simulink model "sm_aileron_actuator_mech_01_ail"  (R2026a)
settings: Solver=VariableStepAuto  EnableMultiTasking=on
PreLoadFcn:
  | aileronAssembly_DataFile
undefined symbols (not defined in the file): AAC_Param, actbase_x, actbase_y, smiData, X, Y, Z
libraries: sm_lib x303, nesl_utility x1
(part 2 of 6)

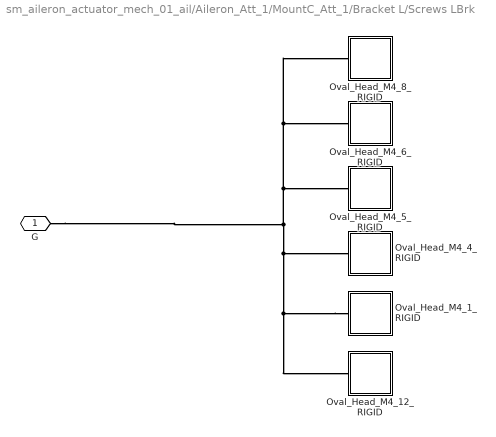
== system sm_aileron_actuator_mech_01_ail/Aileron_Att_1/MountC_Att_1/Bracket L/Screws LBrk ==
  Oval_Head_M4_12_RIGID : Subsystem  RequirementInfo={} %GIDa_408545e4_969e_4b12_8d49_3ebac226240b
  Oval_Head_M4_1_RIGID : Subsystem  RequirementInfo={} %GIDa_fd160c21_93a2_41e0_88bc_776c68d5a1b4
  Oval_Head_M4_4_RIGID : Subsystem  RequirementInfo={} %GIDa_6f4e9814_9943_43be_96b6_78b1aff6dd74
  Oval_Head_M4_5_RIGID : Subsystem  RequirementInfo={} %GIDa_7c459a83_8431_46f1_9d88_31310de40f59
  Oval_Head_M4_6_RIGID : Subsystem  RequirementInfo={} %GIDa_d922eb42_8b80_410e_876a_99bf2bbe6032
  Oval_Head_M4_8_RIGID : Subsystem  RequirementInfo={} %GIDa_ea3f8b8a_bed4_4299_99e1_7a89c2fafe6f
  G : PMIOPort  RequirementInfo={} %GIDa_d90268cf_c8b4_4cb9_9e17_a6888775eb52  Side=Left
  connections:
  Oval_Head_M4_1_RIGID/LConn1 -- G/RConn1 -- Oval_Head_M4_8_RIGID/LConn1 -- Oval_Head_M4_6_RIGID/LConn1 -- Oval_Head_M4_5_RIGID/LConn1 -- Oval_Head_M4_4_RIGID/LConn1 -- Oval_Head_M4_12_RIGID/LConn1

== system sm_aileron_actuator_mech_01_ail/Aileron_Att_1/MountC_Att_1/Bracket R/AilBrk_R_1_RIGID ==
  ReferenceFrame : sm_lib/Frames and Transforms/Reference Frame  RequirementInfo={} %GIDa_74c56975_f3eb_4fd4_b567_ce3850dcc004
  Solid : sm_lib/Body Elements/File Solid  RequirementInfo={} %GIDa_802e2630_df3e_46c3_94a4_2f58f44522fa  ExtGeomFileName=AilBrk_R.step  UnitType=FromFile  ExtGeomFileUnits=m  StepReaderType=HEX  ExportConvexHullGeometry=off  InertiaType=Custom  BasedOnType=Density  Density=1000  DensityUnits=kg/m^3  Mass=smiData.Solid(16).mass  MassUnits=kg  CenterOfMass=smiData.Solid(16).CoM  CenterOfMassUnits=m  MomentsOfInertia=smiData.Solid(16).MoI  MomentsOfInertiaUnits=kg*m^2  ProductsOfInertia=smiData.Solid(16).PoI  ProductsOfInertiaUnits=kg*m^2  GraphicType=FromGeometry  MarkerShape=Sphere  MarkerSize=10  GraphicVisPropType=SimpleVisualProperties  GraphicDiffuseColor=smiData.Solid(16).color  GraphicOpacity=smiData.Solid(16).opacity  GraphicSpecularColor=[0.5 0.5 0.5 1.0]  GraphicAmbientColor=[0.15 0.15 0.15 1.0]  GraphicEmissiveColor=[0.0 0.0 0.0 1.0]  GraphicShininess=75  DoExposeReferenceFrame=on  SerializedFrames=<Frames/>
  Transform : sm_lib/Frames and Transforms/Rigid Transform  RequirementInfo={} %GIDa_83aa15e3_dddf_412e_ac7a_0a1ce9ef137c  RotationMethod=ArbitraryAxis  FollAlignAxisA=+X  BaseAlignAxisA=+Y  FollAlignAxisB=+Y  BaseAlignAxisB=+Z  RotationStandardAxis=+Z  RotationAngle=smiData.RigidTransform(82).angle  RotationAngleUnits=rad  RotationArbitraryAxis=smiData.RigidTransform(82).axis  RotationSequenceAxes=FollowerAxes  RotationSequence=XYX  RotationSequenceAngles=[0 0 0]  RotationSequenceAnglesUnits=deg  RotationMatrix=[1 0 0; 0 1 0; 0 0 1]  Quaternion=[1 0 0 0]  TranslationMethod=Cartesian  TranslationCartesianOffset=smiData.RigidTransform(82).translation  TranslationCartesianOffsetUnits=m  TranslationStandardAxis=+Z  TranslationStandardOffset=0  TranslationStandardOffsetUnits=m  TranslationROffset=0  TranslationROffsetUnits=m  TranslationThetaOffset=0  TranslationThetaOffsetUnits=deg  TranslationZOffset=0  TranslationZOffsetUnits=m
  Transform Manual4Vis : sm_lib/Frames and Transforms/Rigid Transform  RequirementInfo={} %GIDa_283d4460_364a_4cfb_ae13_3c69dcaaddcc  RotationMethod=None  FollAlignAxisA=+X  BaseAlignAxisA=+Y  FollAlignAxisB=+Y  BaseAlignAxisB=+Z  RotationStandardAxis=+Z  RotationAngle=0.0  RotationAngleUnits=deg  RotationArbitraryAxis=[0 0 1]  RotationSequenceAxes=FollowerAxes  RotationSequence=XYX  RotationSequenceAngles=[0 0 0]  RotationSequenceAnglesUnits=deg  RotationMatrix=[1 0 0; 0 1 0; 0 0 1]  Quaternion=[1 0 0 0]  TranslationMethod=StandardAxis  TranslationCartesianOffset=[0 0 0]  TranslationCartesianOffsetUnits=m  TranslationStandardAxis=-Y  TranslationStandardOffset=AAC_Param.AilBrk.LRManual4Vis  TranslationStandardOffsetUnits=m  TranslationROffset=0  TranslationROffsetUnits=m  TranslationThetaOffset=0  TranslationThetaOffsetUnits=deg  TranslationZOffset=0  TranslationZOffsetUnits=m
  Transform1 : sm_lib/Frames and Transforms/Rigid Transform  RequirementInfo={} %GIDa_a1c92bec_f7fd_44f1_b946_6fd160cd1aa4  RotationMethod=ArbitraryAxis  FollAlignAxisA=+X  BaseAlignAxisA=+Y  FollAlignAxisB=+Y  BaseAlignAxisB=+Z  RotationStandardAxis=+Z  RotationAngle=smiData.RigidTransform(176).angle  RotationAngleUnits=rad  RotationArbitraryAxis=smiData.RigidTransform(176).axis  RotationSequenceAxes=FollowerAxes  RotationSequence=XYX  RotationSequenceAngles=[0 0 0]  RotationSequenceAnglesUnits=deg  RotationMatrix=[1 0 0; 0 1 0; 0 0 1]  Quaternion=[1 0 0 0]  TranslationMethod=Cartesian  TranslationCartesianOffset=smiData.RigidTransform(176).translation  TranslationCartesianOffsetUnits=m  TranslationStandardAxis=+Z  TranslationStandardOffset=0  TranslationStandardOffsetUnits=m  TranslationROffset=0  TranslationROffsetUnits=m  TranslationThetaOffset=0  TranslationThetaOffsetUnits=deg  TranslationZOffset=0  TranslationZOffsetUnits=m
  G : PMIOPort  RequirementInfo={} %GIDa_d384faa3_ef63_4569_b23e_5e858ec3c873  Side=Left
  F : PMIOPort  RequirementInfo={} %GIDa_a6f33151_7075_4140_acee_fcb6192613cb  Port=2  Side=Right
  connections:
  Transform Manual4Vis/LConn1 -- ReferenceFrame/RConn1 -- Transform1/LConn1 -- Transform/RConn1
  Transform/LConn1 -- G/RConn1
  Transform1/RConn1 -- F/RConn1
  Transform Manual4Vis/RConn1 -- Solid/RConn1

== system sm_aileron_actuator_mech_01_ail/Aileron_Att_1/MountC_Att_1/Bracket R/Bolt RBrk ==
  Hex_Bolt_M10_1_RIGID : Subsystem  RequirementInfo={} %GIDa_51443a49_e410_4c6d_a840_81d676008002
  Washer_2_RIGID : Subsystem  RequirementInfo={} %GIDa_85bd74db_0059_4442_b071_fa5b0071d56b
  G : PMIOPort  RequirementInfo={} %GIDa_2cce0c68_3112_45a6_92fd_f121ce5f1707  Side=Left
  connections:
  Hex_Bolt_M10_1_RIGID/LConn1 -- G/RConn1 -- Washer_2_RIGID/LConn1

== system sm_aileron_actuator_mech_01_ail/Aileron_Att_1/MountC_Att_1/Bracket R/Screws RBrk ==
  Oval_Head_M4_10_RIGID : Subsystem  RequirementInfo={} %GIDa_d0d1d250_6a18_49bc_9058_b5b8dcd1b587
  Oval_Head_M4_11_RIGID : Subsystem  RequirementInfo={} %GIDa_1e18def3_4770_457a_b532_f3b10f3dd7ac
  Oval_Head_M4_2_RIGID : Subsystem  RequirementInfo={} %GIDa_434c022c_7618_4f4a_9cd7_ab87bc38975f
  Oval_Head_M4_3_RIGID : Subsystem  RequirementInfo={} %GIDa_57ddbddc_0d8f_4cec_bf5d_8c5a1e167ae3
  Oval_Head_M4_7_RIGID : Subsystem  RequirementInfo={} %GIDa_79914485_e7cc_41fb_90bc_5dca6c20becd
  Oval_Head_M4_9_RIGID : Subsystem  RequirementInfo={} %GIDa_ea88f9c1_5feb_464a_844f_15d140c7da09
  G : PMIOPort  RequirementInfo={} %GIDa_a28f78b5_595c_4617_9aa7_5b39891ac86f  Side=Left
  connections:
  Oval_Head_M4_3_RIGID/LConn1 -- G/RConn1 -- Oval_Head_M4_10_RIGID/LConn1 -- Oval_Head_M4_11_RIGID/LConn1 -- Oval_Head_M4_2_RIGID/LConn1 -- Oval_Head_M4_9_RIGID/LConn1 -- Oval_Head_M4_7_RIGID/LConn1

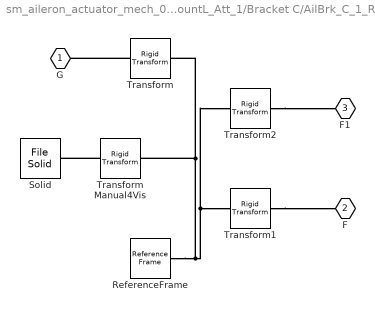
== system sm_aileron_actuator_mech_01_ail/Aileron_Att_1/MountL_Att_1/Bracket C/AilBrk_C_1_RIGID ==
  ReferenceFrame : sm_lib/Frames and Transforms/Reference Frame  RequirementInfo={} %GIDa_a871696a_d055_4df2_9121_142ef3f09b37
  Solid : sm_lib/Body Elements/File Solid  RequirementInfo={} %GIDa_5a36d86e_9075_441a_b790_2426bf56c7da  ExtGeomFileName=AilBrk_C.step  UnitType=FromFile  ExtGeomFileUnits=m  StepReaderType=HEX  ExportConvexHullGeometry=off  InertiaType=Custom  BasedOnType=Density  Density=1000  DensityUnits=kg/m^3  Mass=smiData.Solid(15).mass  MassUnits=kg  CenterOfMass=smiData.Solid(15).CoM  CenterOfMassUnits=m  MomentsOfInertia=smiData.Solid(15).MoI  MomentsOfInertiaUnits=kg*m^2  ProductsOfInertia=smiData.Solid(15).PoI  ProductsOfInertiaUnits=kg*m^2  GraphicType=FromGeometry  MarkerShape=Sphere  MarkerSize=10  GraphicVisPropType=SimpleVisualProperties  GraphicDiffuseColor=smiData.Solid(15).color  GraphicOpacity=smiData.Solid(15).opacity  GraphicSpecularColor=[0.5 0.5 0.5 1.0]  GraphicAmbientColor=[0.15 0.15 0.15 1.0]  GraphicEmissiveColor=[0.0 0.0 0.0 1.0]  GraphicShininess=75  DoExposeReferenceFrame=on  SerializedFrames=<Frames/>
  Transform : sm_lib/Frames and Transforms/Rigid Transform  RequirementInfo={} %GIDa_bf2783ef_b105_4d78_871d_57743bb0bee2  RotationMethod=ArbitraryAxis  FollAlignAxisA=+X  BaseAlignAxisA=+Y  FollAlignAxisB=+Y  BaseAlignAxisB=+Z  RotationStandardAxis=+Z  RotationAngle=smiData.RigidTransform(161).angle  RotationAngleUnits=rad  RotationArbitraryAxis=smiData.RigidTransform(161).axis  RotationSequenceAxes=FollowerAxes  RotationSequence=XYX  RotationSequenceAngles=[0 0 0]  RotationSequenceAnglesUnits=deg  RotationMatrix=[1 0 0; 0 1 0; 0 0 1]  Quaternion=[1 0 0 0]  TranslationMethod=Cartesian  TranslationCartesianOffset=smiData.RigidTransform(161).translation  TranslationCartesianOffsetUnits=m  TranslationStandardAxis=+Z  TranslationStandardOffset=0  TranslationStandardOffsetUnits=m  TranslationROffset=0  TranslationROffsetUnits=m  TranslationThetaOffset=0  TranslationThetaOffsetUnits=deg  TranslationZOffset=0  TranslationZOffsetUnits=m
  Transform Manual4Vis : sm_lib/Frames and Transforms/Rigid Transform  RequirementInfo={} %GIDa_31586e81_9f9a_4547_bcb3_9e99a8f792ea  RotationMethod=None  FollAlignAxisA=+X  BaseAlignAxisA=+Y  FollAlignAxisB=+Y  BaseAlignAxisB=+Z  RotationStandardAxis=+Z  RotationAngle=0.0  RotationAngleUnits=deg  RotationArbitraryAxis=[0 0 1]  RotationSequenceAxes=FollowerAxes  RotationSequence=XYX  RotationSequenceAngles=[0 0 0]  RotationSequenceAnglesUnits=deg  RotationMatrix=[1 0 0; 0 1 0; 0 0 1]  Quaternion=[1 0 0 0]  TranslationMethod=Cartesian  TranslationCartesianOffset=[-1 1 0]*AAC_Param.AilBrk.LRManual4Vis  TranslationCartesianOffsetUnits=m  TranslationStandardAxis=+Z  TranslationStandardOffset=0  TranslationStandardOffsetUnits=m  TranslationROffset=0  TranslationROffsetUnits=m  TranslationThetaOffset=0  TranslationThetaOffsetUnits=deg  TranslationZOffset=0  TranslationZOffsetUnits=m
  Transform1 : sm_lib/Frames and Transforms/Rigid Transform  RequirementInfo={} %GIDa_71a8cba1_f9af_4bc8_a1c0_4002b6347aec  RotationMethod=ArbitraryAxis  FollAlignAxisA=+X  BaseAlignAxisA=+Y  FollAlignAxisB=+Y  BaseAlignAxisB=+Z  RotationStandardAxis=+Z  RotationAngle=smiData.RigidTransform(185).angle  RotationAngleUnits=rad  RotationArbitraryAxis=smiData.RigidTransform(185).axis  RotationSequenceAxes=FollowerAxes  RotationSequence=XYX  RotationSequenceAngles=[0 0 0]  RotationSequenceAnglesUnits=deg  RotationMatrix=[1 0 0; 0 1 0; 0 0 1]  Quaternion=[1 0 0 0]  TranslationMethod=Cartesian  TranslationCartesianOffset=smiData.RigidTransform(185).translation  TranslationCartesianOffsetUnits=m  TranslationStandardAxis=+Z  TranslationStandardOffset=0  TranslationStandardOffsetUnits=m  TranslationROffset=0  TranslationROffsetUnits=m  TranslationThetaOffset=0  TranslationThetaOffsetUnits=deg  TranslationZOffset=0  TranslationZOffsetUnits=m
  Transform2 : sm_lib/Frames and Transforms/Rigid Transform  RequirementInfo={} %GIDa_2e2375df_b38c_4b24_9016_3885bd582684  RotationMethod=ArbitraryAxis  FollAlignAxisA=+X  BaseAlignAxisA=+Y  FollAlignAxisB=+Y  BaseAlignAxisB=+Z  RotationStandardAxis=+Z  RotationAngle=smiData.RigidTransform(202).angle  RotationAngleUnits=rad  RotationArbitraryAxis=smiData.RigidTransform(202).axis  RotationSequenceAxes=FollowerAxes  RotationSequence=XYX  RotationSequenceAngles=[0 0 0]  RotationSequenceAnglesUnits=deg  RotationMatrix=[1 0 0; 0 1 0; 0 0 1]  Quaternion=[1 0 0 0]  TranslationMethod=Cartesian  TranslationCartesianOffset=smiData.RigidTransform(202).translation  TranslationCartesianOffsetUnits=m  TranslationStandardAxis=+Z  TranslationStandardOffset=0  TranslationStandardOffsetUnits=m  TranslationROffset=0  TranslationROffsetUnits=m  TranslationThetaOffset=0  TranslationThetaOffsetUnits=deg  TranslationZOffset=0  TranslationZOffsetUnits=m
  G : PMIOPort  RequirementInfo={} %GIDa_7e064869_dbf4_4faa_9353_bbd675a5631f  Side=Left
  F : PMIOPort  RequirementInfo={} %GIDa_0afa8f43_6a7a_4b49_b07b_aff7a5ad6afd  Port=2  Side=Right
  F1 : PMIOPort  RequirementInfo={} %GIDa_f0cc7407_108c_42b1_8ac8_baa841156f5e  Port=3  Side=Left
  connections:
  Transform Manual4Vis/LConn1 -- ReferenceFrame/RConn1 -- Transform1/LConn1 -- Transform2/LConn1 -- Transform/RConn1
  Transform/LConn1 -- G/RConn1
  Transform1/RConn1 -- F/RConn1
  Transform2/RConn1 -- F1/RConn1
  Transform Manual4Vis/RConn1 -- Solid/RConn1

== system sm_aileron_actuator_mech_01_ail/Aileron_Att_1/MountL_Att_1/Bracket C/Bolt CBrk ==
  Hex_Bolt_M10_3_RIGID : Subsystem  RequirementInfo={} %GIDa_38a28924_e615_4e04_ad8c_1e483bc2f21f
  Hex_Flange_Nut_M10_1_RIGID : Subsystem  RequirementInfo={} %GIDa_5164e672_dad8_4f4b_8ea6_9a1e87213717
  Washer_1_RIGID : Subsystem  RequirementInfo={} %GIDa_764df6da_276f_4ad9_844d_4a9a6a6437d3
  Washer_4_RIGID : Subsystem  RequirementInfo={} %GIDa_7d7c93c2_0cd1_4f9f_9a94_ccd0146b44b1
  G : PMIOPort  RequirementInfo={} %GIDa_84dc20b9_d51f_4cb9_961c_d7f22f1421d3  Side=Left
  connections:
  Hex_Flange_Nut_M10_1_RIGID/LConn1 -- G/RConn1 -- Hex_Bolt_M10_3_RIGID/LConn1 -- Washer_1_RIGID/LConn1 -- Washer_4_RIGID/LConn1

== system sm_aileron_actuator_mech_01_ail/Aileron_Att_1/MountL_Att_1/Bracket C/Screws CBrk ==
  Hex_Flange_Screw_M6_1_RIGID : Subsystem  RequirementInfo={} %GIDa_57cbeea6_7533_4ae1_b6e6_370846aff067
  Hex_Flange_Screw_M6_2_RIGID : Subsystem  RequirementInfo={} %GIDa_27bd2fbe_9c91_404e_ae7b_ecc53260d8de
  Hex_Flange_Screw_M6_3_RIGID : Subsystem  RequirementInfo={} %GIDa_e4d2040f_bb89_4ea2_b766_68c73890896b
  Hex_Flange_Screw_M6_4_RIGID : Subsystem  RequirementInfo={} %GIDa_9c69fd48_7898_47d5_9f24_7ecd9bf76219
  Hex_Flange_Screw_M6_5_RIGID : Subsystem  RequirementInfo={} %GIDa_20e62b24_5f2a_4870_a79a_ec0ec785b89b
  Hex_Flange_Screw_M6_6_RIGID : Subsystem  RequirementInfo={} %GIDa_e7d78725_d01c_420c_b848_1ea210de75ca
  G : PMIOPort  RequirementInfo={} %GIDa_07c51d8b_11c1_4822_a9ed_4dbaf68434e2  Side=Left
  connections:
  Hex_Flange_Screw_M6_6_RIGID/LConn1 -- G/RConn1 -- Hex_Flange_Screw_M6_1_RIGID/LConn1 -- Hex_Flange_Screw_M6_2_RIGID/LConn1 -- Hex_Flange_Screw_M6_3_RIGID/LConn1 -- Hex_Flange_Screw_M6_4_RIGID/LConn1 -- Hex_Flange_Screw_M6_5_RIGID/LConn1

== system sm_aileron_actuator_mech_01_ail/Aileron_Att_1/MountL_Att_1/Bracket L/AilBrk_L_1_RIGID ==
  ReferenceFrame : sm_lib/Frames and Transforms/Reference Frame  RequirementInfo={} %GIDa_39332f9b_e32f_409e_9b4b_dabf2a0a1018
  Solid : sm_lib/Body Elements/File Solid  RequirementInfo={} %GIDa_11a5346b_4455_4e0f_aa01_5f22ff06b31e  ExtGeomFileName=AilBrk_L.step  UnitType=FromFile  ExtGeomFileUnits=m  StepReaderType=HEX  ExportConvexHullGeometry=off  InertiaType=Custom  BasedOnType=Density  Density=1000  DensityUnits=kg/m^3  Mass=smiData.Solid(13).mass  MassUnits=kg  CenterOfMass=smiData.Solid(13).CoM  CenterOfMassUnits=m  MomentsOfInertia=smiData.Solid(13).MoI  MomentsOfInertiaUnits=kg*m^2  ProductsOfInertia=smiData.Solid(13).PoI  ProductsOfInertiaUnits=kg*m^2  GraphicType=FromGeometry  MarkerShape=Sphere  MarkerSize=10  GraphicVisPropType=SimpleVisualProperties  GraphicDiffuseColor=smiData.Solid(13).color  GraphicOpacity=smiData.Solid(13).opacity  GraphicSpecularColor=[0.5 0.5 0.5 1.0]  GraphicAmbientColor=[0.15 0.15 0.15 1.0]  GraphicEmissiveColor=[0.0 0.0 0.0 1.0]  GraphicShininess=75  DoExposeReferenceFrame=on  SerializedFrames=<Frames/>
  Transform : sm_lib/Frames and Transforms/Rigid Transform  RequirementInfo={} %GIDa_5daa17ec_3b60_44a1_9561_92beb52b62cc  RotationMethod=ArbitraryAxis  FollAlignAxisA=+X  BaseAlignAxisA=+Y  FollAlignAxisB=+Y  BaseAlignAxisB=+Z  RotationStandardAxis=+Z  RotationAngle=smiData.RigidTransform(150).angle  RotationAngleUnits=rad  RotationArbitraryAxis=smiData.RigidTransform(150).axis  RotationSequenceAxes=FollowerAxes  RotationSequence=XYX  RotationSequenceAngles=[0 0 0]  RotationSequenceAnglesUnits=deg  RotationMatrix=[1 0 0; 0 1 0; 0 0 1]  Quaternion=[1 0 0 0]  TranslationMethod=Cartesian  TranslationCartesianOffset=smiData.RigidTransform(150).translation  TranslationCartesianOffsetUnits=m  TranslationStandardAxis=+Z  TranslationStandardOffset=0  TranslationStandardOffsetUnits=m  TranslationROffset=0  TranslationROffsetUnits=m  TranslationThetaOffset=0  TranslationThetaOffsetUnits=deg  TranslationZOffset=0  TranslationZOffsetUnits=m
  Transform Manual4Vis : sm_lib/Frames and Transforms/Rigid Transform  RequirementInfo={} %GIDa_5a6217b2_7528_4058_aa54_b4f74b02c073  RotationMethod=None  FollAlignAxisA=+X  BaseAlignAxisA=+Y  FollAlignAxisB=+Y  BaseAlignAxisB=+Z  RotationStandardAxis=+Z  RotationAngle=0.0  RotationAngleUnits=deg  RotationArbitraryAxis=[0 0 1]  RotationSequenceAxes=FollowerAxes  RotationSequence=XYX  RotationSequenceAngles=[0 0 0]  RotationSequenceAnglesUnits=deg  RotationMatrix=[1 0 0; 0 1 0; 0 0 1]  Quaternion=[1 0 0 0]  TranslationMethod=StandardAxis  TranslationCartesianOffset=[0 0 0]  TranslationCartesianOffsetUnits=m  TranslationStandardAxis=+Y  TranslationStandardOffset=AAC_Param.AilBrk.LRManual4Vis  TranslationStandardOffsetUnits=m  TranslationROffset=0  TranslationROffsetUnits=m  TranslationThetaOffset=0  TranslationThetaOffsetUnits=deg  TranslationZOffset=0  TranslationZOffsetUnits=m
  Transform1 : sm_lib/Frames and Transforms/Rigid Transform  RequirementInfo={} %GIDa_822542f5_65e6_411d_8362_1ca7be96dec1  RotationMethod=ArbitraryAxis  FollAlignAxisA=+X  BaseAlignAxisA=+Y  FollAlignAxisB=+Y  BaseAlignAxisB=+Z  RotationStandardAxis=+Z  RotationAngle=smiData.RigidTransform(183).angle  RotationAngleUnits=rad  RotationArbitraryAxis=smiData.RigidTransform(183).axis  RotationSequenceAxes=FollowerAxes  RotationSequence=XYX  RotationSequenceAngles=[0 0 0]  RotationSequenceAnglesUnits=deg  RotationMatrix=[1 0 0; 0 1 0; 0 0 1]  Quaternion=[1 0 0 0]  TranslationMethod=Cartesian  TranslationCartesianOffset=smiData.RigidTransform(183).translation  TranslationCartesianOffsetUnits=m  TranslationStandardAxis=+Z  TranslationStandardOffset=0  TranslationStandardOffsetUnits=m  TranslationROffset=0  TranslationROffsetUnits=m  TranslationThetaOffset=0  TranslationThetaOffsetUnits=deg  TranslationZOffset=0  TranslationZOffsetUnits=m
  G : PMIOPort  RequirementInfo={} %GIDa_2653e6de_e41d_49da_bac7_b51017c466e9  Side=Left
  F : PMIOPort  RequirementInfo={} %GIDa_eaf60001_bcca_436a_a8c5_26ad81a65e44  Port=2  Side=Right
  connections:
  Transform Manual4Vis/LConn1 -- ReferenceFrame/RConn1 -- Transform1/LConn1 -- Transform/RConn1
  Transform/LConn1 -- G/RConn1
  Transform1/RConn1 -- F/RConn1
  Transform Manual4Vis/RConn1 -- Solid/RConn1

== system sm_aileron_actuator_mech_01_ail/Aileron_Att_1/MountL_Att_1/Bracket L/Bolt LBrk ==
  Hex_Bolt_M10_1_RIGID : Subsystem  RequirementInfo={} %GIDa_4e318ed6_ee86_4a24_ad7a_90e821571c1d
  Washer_3_RIGID : Subsystem  RequirementInfo={} %GIDa_cf68110c_dbb4_4cf4_b249_e2932fedd0f0
  G : PMIOPort  RequirementInfo={} %GIDa_705a3d34_e05c_491c_91b6_3afc310e1f0c  Side=Left
  connections:
  Washer_3_RIGID/LConn1 -- G/RConn1 -- Hex_Bolt_M10_1_RIGID/LConn1

== system sm_aileron_actuator_mech_01_ail/Aileron_Att_1/MountL_Att_1/Bracket L/Screws LBrk  ==
  Oval_Head_M4_2_RIGID : Subsystem  RequirementInfo={} %GIDa_6c8e6134_23a2_4146_8d12_cda11073c2d6
  Oval_Head_M4_3_RIGID : Subsystem  RequirementInfo={} %GIDa_b68226d0_c2ee_4daa_9115_f885e7707d40
  Oval_Head_M4_4_RIGID : Subsystem  RequirementInfo={} %GIDa_a17d6292_0107_4a69_988a_427b2d012b8d
  Oval_Head_M4_5_RIGID : Subsystem  RequirementInfo={} %GIDa_2e07ecc8_5ef7_49ec_9d50_12f246f43098
  Oval_Head_M4_7_RIGID : Subsystem  RequirementInfo={} %GIDa_1d2ba71d_66cf_4826_955d_272def03ab14
  Oval_Head_M4_9_RIGID : Subsystem  RequirementInfo={} %GIDa_1918bcf2_b04f_41e0_bb07_aca5d7d41cb8
  G : PMIOPort  RequirementInfo={} %GIDa_0e9749be_2295_416c_ae85_6fcf2420ccb5  Side=Left
  connections:
  Oval_Head_M4_9_RIGID/LConn1 -- Oval_Head_M4_7_RIGID/LConn1 -- G/RConn1 -- Oval_Head_M4_2_RIGID/LConn1 -- Oval_Head_M4_3_RIGID/LConn1 -- Oval_Head_M4_4_RIGID/LConn1 -- Oval_Head_M4_5_RIGID/LConn1

== system sm_aileron_actuator_mech_01_ail/Aileron_Att_1/MountL_Att_1/Bracket R/AilBrk_R_1_RIGID ==
  ReferenceFrame : sm_lib/Frames and Transforms/Reference Frame  RequirementInfo={} %GIDa_fda6c982_ec10_46ec_99ba_af4923b682fa
  Solid : sm_lib/Body Elements/File Solid  RequirementInfo={} %GIDa_e72296d1_5341_48ae_bb81_159c83b7f05b  ExtGeomFileName=AilBrk_R.step  UnitType=FromFile  ExtGeomFileUnits=m  StepReaderType=HEX  ExportConvexHullGeometry=off  InertiaType=Custom  BasedOnType=Density  Density=1000  DensityUnits=kg/m^3  Mass=smiData.Solid(16).mass  MassUnits=kg  CenterOfMass=smiData.Solid(16).CoM  CenterOfMassUnits=m  MomentsOfInertia=smiData.Solid(16).MoI  MomentsOfInertiaUnits=kg*m^2  ProductsOfInertia=smiData.Solid(16).PoI  ProductsOfInertiaUnits=kg*m^2  GraphicType=FromGeometry  MarkerShape=Sphere  MarkerSize=10  GraphicVisPropType=SimpleVisualProperties  GraphicDiffuseColor=smiData.Solid(16).color  GraphicOpacity=smiData.Solid(16).opacity  GraphicSpecularColor=[0.5 0.5 0.5 1.0]  GraphicAmbientColor=[0.15 0.15 0.15 1.0]  GraphicEmissiveColor=[0.0 0.0 0.0 1.0]  GraphicShininess=75  DoExposeReferenceFrame=on  SerializedFrames=<Frames/>
  Transform : sm_lib/Frames and Transforms/Rigid Transform  RequirementInfo={} %GIDa_c9ec10d3_2d70_43b2_9623_1faba3e799f1  RotationMethod=ArbitraryAxis  FollAlignAxisA=+X  BaseAlignAxisA=+Y  FollAlignAxisB=+Y  BaseAlignAxisB=+Z  RotationStandardAxis=+Z  RotationAngle=smiData.RigidTransform(146).angle  RotationAngleUnits=rad  RotationArbitraryAxis=smiData.RigidTransform(146).axis  RotationSequenceAxes=FollowerAxes  RotationSequence=XYX  RotationSequenceAngles=[0 0 0]  RotationSequenceAnglesUnits=deg  RotationMatrix=[1 0 0; 0 1 0; 0 0 1]  Quaternion=[1 0 0 0]  TranslationMethod=Cartesian  TranslationCartesianOffset=smiData.RigidTransform(146).translation  TranslationCartesianOffsetUnits=m  TranslationStandardAxis=+Z  TranslationStandardOffset=0  TranslationStandardOffsetUnits=m  TranslationROffset=0  TranslationROffsetUnits=m  TranslationThetaOffset=0  TranslationThetaOffsetUnits=deg  TranslationZOffset=0  TranslationZOffsetUnits=m
  Transform Manual4Vis : sm_lib/Frames and Transforms/Rigid Transform  RequirementInfo={} %GIDa_9229ddc2_51c0_49a4_acef_e04dff0661c7  RotationMethod=None  FollAlignAxisA=+X  BaseAlignAxisA=+Y  FollAlignAxisB=+Y  BaseAlignAxisB=+Z  RotationStandardAxis=+Z  RotationAngle=0.0  RotationAngleUnits=deg  RotationArbitraryAxis=[0 0 1]  RotationSequenceAxes=FollowerAxes  RotationSequence=XYX  RotationSequenceAngles=[0 0 0]  RotationSequenceAnglesUnits=deg  RotationMatrix=[1 0 0; 0 1 0; 0 0 1]  Quaternion=[1 0 0 0]  TranslationMethod=StandardAxis  TranslationCartesianOffset=[0 0 0]  TranslationCartesianOffsetUnits=m  TranslationStandardAxis=-Y  TranslationStandardOffset=AAC_Param.AilBrk.LRManual4Vis  TranslationStandardOffsetUnits=m  TranslationROffset=0  TranslationROffsetUnits=m  TranslationThetaOffset=0  TranslationThetaOffsetUnits=deg  TranslationZOffset=0  TranslationZOffsetUnits=m
  Transform1 : sm_lib/Frames and Transforms/Rigid Transform  RequirementInfo={} %GIDa_1d7f1286_6369_4b86_808f_b629ccc1ba07  RotationMethod=ArbitraryAxis  FollAlignAxisA=+X  BaseAlignAxisA=+Y  FollAlignAxisB=+Y  BaseAlignAxisB=+Z  RotationStandardAxis=+Z  RotationAngle=smiData.RigidTransform(187).angle  RotationAngleUnits=rad  RotationArbitraryAxis=smiData.RigidTransform(187).axis  RotationSequenceAxes=FollowerAxes  RotationSequence=XYX  RotationSequenceAngles=[0 0 0]  RotationSequenceAnglesUnits=deg  RotationMatrix=[1 0 0; 0 1 0; 0 0 1]  Quaternion=[1 0 0 0]  TranslationMethod=Cartesian  TranslationCartesianOffset=smiData.RigidTransform(187).translation  TranslationCartesianOffsetUnits=m  TranslationStandardAxis=+Z  TranslationStandardOffset=0  TranslationStandardOffsetUnits=m  TranslationROffset=0  TranslationROffsetUnits=m  TranslationThetaOffset=0  TranslationThetaOffsetUnits=deg  TranslationZOffset=0  TranslationZOffsetUnits=m
  G : PMIOPort  RequirementInfo={} %GIDa_0bdcb0aa_0fa2_444f_bfc5_3a1bc4dd49f3  Side=Left
  F : PMIOPort  RequirementInfo={} %GIDa_92bad992_680c_4f13_81f1_0f379d9be367  Port=2  Side=Right
  connections:
  Transform Manual4Vis/RConn1 -- Solid/RConn1
  Transform/LConn1 -- G/RConn1
  Transform1/RConn1 -- F/RConn1
  ReferenceFrame/RConn1 -- Transform Manual4Vis/LConn1 -- Transform/RConn1 -- Transform1/LConn1

== system sm_aileron_actuator_mech_01_ail/Aileron_Att_1/MountL_Att_1/Bracket R/Bolt RBrk ==
  Hex_Bolt_M10_2_RIGID : Subsystem  RequirementInfo={} %GIDa_0ecb3382_5d44_4145_9740_8c33c133f781
  Washer_2_RIGID : Subsystem  RequirementInfo={} %GIDa_c53d5f88_06af_49ae_ba86_a081237bfbcc
  G : PMIOPort  RequirementInfo={} %GIDa_9f55d692_4792_4ce0_b96e_7e6d804409a6  Side=Left
  connections:
  G/RConn1 -- Washer_2_RIGID/LConn1 -- Hex_Bolt_M10_2_RIGID/LConn1

== system sm_aileron_actuator_mech_01_ail/Aileron_Att_1/MountL_Att_1/Bracket R/Screws RBrk ==
  Oval_Head_M4_10_RIGID : Subsystem  RequirementInfo={} %GIDa_5bb18d23_377a_4f6b_960f_02d4b23eac72
  Oval_Head_M4_11_RIGID : Subsystem  RequirementInfo={} %GIDa_7614a5d3_d245_4db9_a67f_5827d2586359
  Oval_Head_M4_12_RIGID : Subsystem  RequirementInfo={} %GIDa_cd110108_66ae_4762_b94e_83481f002135
  Oval_Head_M4_1_RIGID : Subsystem  RequirementInfo={} %GIDa_13967627_79ac_470c_86d0_385ede8b0fde
  Oval_Head_M4_6_RIGID : Subsystem  RequirementInfo={} %GIDa_7bee348b_b0b9_4439_ac01_079487ded313
  Oval_Head_M4_8_RIGID : Subsystem  RequirementInfo={} %GIDa_41a8bba5_d613_4361_896e_90222ae71f92
  G : PMIOPort  RequirementInfo={} %GIDa_1fc2baee_654a_4057_8681_e880c71c2f50  Side=Left
  connections:
  Oval_Head_M4_6_RIGID/LConn1 -- G/RConn1 -- Oval_Head_M4_10_RIGID/LConn1 -- Oval_Head_M4_11_RIGID/LConn1 -- Oval_Head_M4_12_RIGID/LConn1 -- Oval_Head_M4_1_RIGID/LConn1 -- Oval_Head_M4_8_RIGID/LConn1

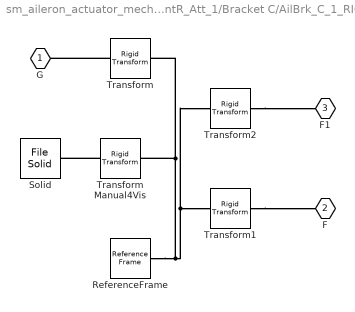
== system sm_aileron_actuator_mech_01_ail/Aileron_Att_1/MountR_Att_1/Bracket C/AilBrk_C_1_RIGID ==
  ReferenceFrame : sm_lib/Frames and Transforms/Reference Frame  RequirementInfo={} %GIDa_d14b405c_5e57_429c_9b86_ffc29183a72f
  Solid : sm_lib/Body Elements/File Solid  RequirementInfo={} %GIDa_4b043c83_956d_4225_8b32_89ad7c693e63  ExtGeomFileName=AilBrk_C.step  UnitType=FromFile  ExtGeomFileUnits=m  StepReaderType=HEX  ExportConvexHullGeometry=off  InertiaType=Custom  BasedOnType=Density  Density=1000  DensityUnits=kg/m^3  Mass=smiData.Solid(15).mass  MassUnits=kg  CenterOfMass=smiData.Solid(15).CoM  CenterOfMassUnits=m  MomentsOfInertia=smiData.Solid(15).MoI  MomentsOfInertiaUnits=kg*m^2  ProductsOfInertia=smiData.Solid(15).PoI  ProductsOfInertiaUnits=kg*m^2  GraphicType=FromGeometry  MarkerShape=Sphere  MarkerSize=10  GraphicVisPropType=SimpleVisualProperties  GraphicDiffuseColor=smiData.Solid(15).color  GraphicOpacity=smiData.Solid(15).opacity  GraphicSpecularColor=[0.5 0.5 0.5 1.0]  GraphicAmbientColor=[0.15 0.15 0.15 1.0]  GraphicEmissiveColor=[0.0 0.0 0.0 1.0]  GraphicShininess=75  DoExposeReferenceFrame=on  SerializedFrames=<Frames/>
  Transform : sm_lib/Frames and Transforms/Rigid Transform  RequirementInfo={} %GIDa_dae4c9e1_5186_464d_af5e_7438ac99136e  RotationMethod=ArbitraryAxis  FollAlignAxisA=+X  BaseAlignAxisA=+Y  FollAlignAxisB=+Y  BaseAlignAxisB=+Z  RotationStandardAxis=+Z  RotationAngle=smiData.RigidTransform(136).angle  RotationAngleUnits=rad  RotationArbitraryAxis=smiData.RigidTransform(136).axis  RotationSequenceAxes=FollowerAxes  RotationSequence=XYX  RotationSequenceAngles=[0 0 0]  RotationSequenceAnglesUnits=deg  RotationMatrix=[1 0 0; 0 1 0; 0 0 1]  Quaternion=[1 0 0 0]  TranslationMethod=Cartesian  TranslationCartesianOffset=smiData.RigidTransform(136).translation  TranslationCartesianOffsetUnits=m  TranslationStandardAxis=+Z  TranslationStandardOffset=0  TranslationStandardOffsetUnits=m  TranslationROffset=0  TranslationROffsetUnits=m  TranslationThetaOffset=0  TranslationThetaOffsetUnits=deg  TranslationZOffset=0  TranslationZOffsetUnits=m
  Transform Manual4Vis : sm_lib/Frames and Transforms/Rigid Transform  RequirementInfo={} %GIDa_fc6156f6_267d_435d_a44d_8024c895094e  RotationMethod=None  FollAlignAxisA=+X  BaseAlignAxisA=+Y  FollAlignAxisB=+Y  BaseAlignAxisB=+Z  RotationStandardAxis=+Z  RotationAngle=0.0  RotationAngleUnits=deg  RotationArbitraryAxis=[0 0 1]  RotationSequenceAxes=FollowerAxes  RotationSequence=XYX  RotationSequenceAngles=[0 0 0]  RotationSequenceAnglesUnits=deg  RotationMatrix=[1 0 0; 0 1 0; 0 0 1]  Quaternion=[1 0 0 0]  TranslationMethod=Cartesian  TranslationCartesianOffset=[-1 1 0]*AAC_Param.AilBrk.LRManual4Vis  TranslationCartesianOffsetUnits=m  TranslationStandardAxis=+Z  TranslationStandardOffset=0  TranslationStandardOffsetUnits=m  TranslationROffset=0  TranslationROffsetUnits=m  TranslationThetaOffset=0  TranslationThetaOffsetUnits=deg  TranslationZOffset=0  TranslationZOffsetUnits=m
  Transform1 : sm_lib/Frames and Transforms/Rigid Transform  RequirementInfo={} %GIDa_835145d4_0c58_474f_8a7d_93398a0ecc3e  RotationMethod=ArbitraryAxis  FollAlignAxisA=+X  BaseAlignAxisA=+Y  FollAlignAxisB=+Y  BaseAlignAxisB=+Z  RotationStandardAxis=+Z  RotationAngle=smiData.RigidTransform(181).angle  RotationAngleUnits=rad  RotationArbitraryAxis=smiData.RigidTransform(181).axis  RotationSequenceAxes=FollowerAxes  RotationSequence=XYX  RotationSequenceAngles=[0 0 0]  RotationSequenceAnglesUnits=deg  RotationMatrix=[1 0 0; 0 1 0; 0 0 1]  Quaternion=[1 0 0 0]  TranslationMethod=Cartesian  TranslationCartesianOffset=smiData.RigidTransform(181).translation  TranslationCartesianOffsetUnits=m  TranslationStandardAxis=+Z  TranslationStandardOffset=0  TranslationStandardOffsetUnits=m  TranslationROffset=0  TranslationROffsetUnits=m  TranslationThetaOffset=0  TranslationThetaOffsetUnits=deg  TranslationZOffset=0  TranslationZOffsetUnits=m
  Transform2 : sm_lib/Frames and Transforms/Rigid Transform  RequirementInfo={} %GIDa_3625548a_86dd_49d3_a897_69214354849c  RotationMethod=ArbitraryAxis  FollAlignAxisA=+X  BaseAlignAxisA=+Y  FollAlignAxisB=+Y  BaseAlignAxisB=+Z  RotationStandardAxis=+Z  RotationAngle=smiData.RigidTransform(192).angle  RotationAngleUnits=rad  RotationArbitraryAxis=smiData.RigidTransform(192).axis  RotationSequenceAxes=FollowerAxes  RotationSequence=XYX  RotationSequenceAngles=[0 0 0]  RotationSequenceAnglesUnits=deg  RotationMatrix=[1 0 0; 0 1 0; 0 0 1]  Quaternion=[1 0 0 0]  TranslationMethod=Cartesian  TranslationCartesianOffset=smiData.RigidTransform(192).translation  TranslationCartesianOffsetUnits=m  TranslationStandardAxis=+Z  TranslationStandardOffset=0  TranslationStandardOffsetUnits=m  TranslationROffset=0  TranslationROffsetUnits=m  TranslationThetaOffset=0  TranslationThetaOffsetUnits=deg  TranslationZOffset=0  TranslationZOffsetUnits=m
  G : PMIOPort  RequirementInfo={} %GIDa_fb90886c_5768_4895_8fea_0b7b08e07bb2  Side=Left
  F : PMIOPort  RequirementInfo={} %GIDa_c0d10456_7555_4e9b_bf84_d7440f84960b  Port=2  Side=Right
  F1 : PMIOPort  RequirementInfo={} %GIDa_ce2d166f_d5b6_4794_91e8_9365d27cbe97  Port=3  Side=Left
  connections:
  Transform Manual4Vis/LConn1 -- ReferenceFrame/RConn1 -- Transform1/LConn1 -- Transform2/LConn1 -- Transform/RConn1
  Transform/LConn1 -- G/RConn1
  Transform1/RConn1 -- F/RConn1
  Transform2/RConn1 -- F1/RConn1
  Transform Manual4Vis/RConn1 -- Solid/RConn1

== system sm_aileron_actuator_mech_01_ail/Aileron_Att_1/MountR_Att_1/Bracket C/Bolt CBrk ==
  Hex_Bolt_M10_3_RIGID : Subsystem  RequirementInfo={} %GIDa_19303b2e_db77_424e_9eb1_61ed69e6e753
  Hex_Flange_Nut_M10_1_RIGID : Subsystem  RequirementInfo={} %GIDa_d88d2036_979f_4a20_97ee_41d3ee39d431
  Washer_2_RIGID : Subsystem  RequirementInfo={} %GIDa_9de33c89_bb74_441d_8dac_61b3e05ae3c4
  Washer_4_RIGID : Subsystem  RequirementInfo={} %GIDa_2a1dfb8b_250a_4f5c_8075_7a8b180174d8
  B : PMIOPort  RequirementInfo={} %GIDa_ca1d19f8_aa8b_478a_af36_84b24160058b  Side=Left
  connections:
  Washer_4_RIGID/LConn1 -- B/RConn1 -- Washer_2_RIGID/LConn1 -- Hex_Flange_Nut_M10_1_RIGID/LConn1 -- Hex_Bolt_M10_3_RIGID/LConn1

== system sm_aileron_actuator_mech_01_ail/Aileron_Att_1/MountR_Att_1/Bracket C/Screws CBrk ==
  Hex_Flange_Screw_M6_1_RIGID : Subsystem  RequirementInfo={} %GIDa_d41f617b_d13a_473c_aefc_1ccebdadc082
  Hex_Flange_Screw_M6_2_RIGID : Subsystem  RequirementInfo={} %GIDa_3197cadb_a000_4ab6_b1a7_844c5839960c
  Hex_Flange_Screw_M6_3_RIGID : Subsystem  RequirementInfo={} %GIDa_51ce801b_a5f2_468a_9b5e_272bd336ffc4
  Hex_Flange_Screw_M6_4_RIGID : Subsystem  RequirementInfo={} %GIDa_cf1f4249_3965_4ff9_ac1a_f8ef4bb7a97d
  Hex_Flange_Screw_M6_5_RIGID : Subsystem  RequirementInfo={} %GIDa_9e29edf0_c5fb_4f8e_9bf1_14024b8b5ed9
  Hex_Flange_Screw_M6_6_RIGID : Subsystem  RequirementInfo={} %GIDa_9f631fec_403c_4f5e_afca_52e077f3d381
  B : PMIOPort  RequirementInfo={} %GIDa_6e731daa_665a_4d35_81e5_70a24f5ce88e  Side=Left
  connections:
  B/RConn1 -- Hex_Flange_Screw_M6_6_RIGID/LConn1 -- Hex_Flange_Screw_M6_5_RIGID/LConn1 -- Hex_Flange_Screw_M6_4_RIGID/LConn1 -- Hex_Flange_Screw_M6_3_RIGID/LConn1 -- Hex_Flange_Screw_M6_2_RIGID/LConn1 -- Hex_Flange_Screw_M6_1_RIGID/LConn1

== system sm_aileron_actuator_mech_01_ail/Aileron_Att_1/MountR_Att_1/Bracket L/AilBrk_L_1_RIGID ==
  ReferenceFrame : sm_lib/Frames and Transforms/Reference Frame  RequirementInfo={} %GIDa_9cd44e07_ab93_4d71_a2f1_75686e4286f3
  Solid : sm_lib/Body Elements/File Solid  RequirementInfo={} %GIDa_3ec32f81_ed25_4796_a0b4_d9763d76a1cc  ExtGeomFileName=AilBrk_L.step  UnitType=FromFile  ExtGeomFileUnits=m  StepReaderType=HEX  ExportConvexHullGeometry=off  InertiaType=Custom  BasedOnType=Density  Density=1000  DensityUnits=kg/m^3  Mass=smiData.Solid(13).mass  MassUnits=kg  CenterOfMass=smiData.Solid(13).CoM  CenterOfMassUnits=m  MomentsOfInertia=smiData.Solid(13).MoI  MomentsOfInertiaUnits=kg*m^2  ProductsOfInertia=smiData.Solid(13).PoI  ProductsOfInertiaUnits=kg*m^2  GraphicType=FromGeometry  MarkerShape=Sphere  MarkerSize=10  GraphicVisPropType=SimpleVisualProperties  GraphicDiffuseColor=smiData.Solid(13).color  GraphicOpacity=smiData.Solid(13).opacity  GraphicSpecularColor=[0.5 0.5 0.5 1.0]  GraphicAmbientColor=[0.15 0.15 0.15 1.0]  GraphicEmissiveColor=[0.0 0.0 0.0 1.0]  GraphicShininess=75  DoExposeReferenceFrame=on  SerializedFrames=<Frames/>
  Transform : sm_lib/Frames and Transforms/Rigid Transform  RequirementInfo={} %GIDa_2ad5d089_0c1e_4b22_886f_a5bac31088d3  RotationMethod=ArbitraryAxis  FollAlignAxisA=+X  BaseAlignAxisA=+Y  FollAlignAxisB=+Y  BaseAlignAxisB=+Z  RotationStandardAxis=+Z  RotationAngle=smiData.RigidTransform(116).angle  RotationAngleUnits=rad  RotationArbitraryAxis=smiData.RigidTransform(116).axis  RotationSequenceAxes=FollowerAxes  RotationSequence=XYX  RotationSequenceAngles=[0 0 0]  RotationSequenceAnglesUnits=deg  RotationMatrix=[1 0 0; 0 1 0; 0 0 1]  Quaternion=[1 0 0 0]  TranslationMethod=Cartesian  TranslationCartesianOffset=smiData.RigidTransform(116).translation  TranslationCartesianOffsetUnits=m  TranslationStandardAxis=+Z  TranslationStandardOffset=0  TranslationStandardOffsetUnits=m  TranslationROffset=0  TranslationROffsetUnits=m  TranslationThetaOffset=0  TranslationThetaOffsetUnits=deg  TranslationZOffset=0  TranslationZOffsetUnits=m
  Transform Manual4Vis : sm_lib/Frames and Transforms/Rigid Transform  RequirementInfo={} %GIDa_773760b3_ce08_42aa_ab71_6ee1f7d5b109  RotationMethod=None  FollAlignAxisA=+X  BaseAlignAxisA=+Y  FollAlignAxisB=+Y  BaseAlignAxisB=+Z  RotationStandardAxis=+Z  RotationAngle=0.0  RotationAngleUnits=deg  RotationArbitraryAxis=[0 0 1]  RotationSequenceAxes=FollowerAxes  RotationSequence=XYX  RotationSequenceAngles=[0 0 0]  RotationSequenceAnglesUnits=deg  RotationMatrix=[1 0 0; 0 1 0; 0 0 1]  Quaternion=[1 0 0 0]  TranslationMethod=StandardAxis  TranslationCartesianOffset=[0 0 0]  TranslationCartesianOffsetUnits=m  TranslationStandardAxis=+Y  TranslationStandardOffset=AAC_Param.AilBrk.LRManual4Vis  TranslationStandardOffsetUnits=m  TranslationROffset=0  TranslationROffsetUnits=m  TranslationThetaOffset=0  TranslationThetaOffsetUnits=deg  TranslationZOffset=0  TranslationZOffsetUnits=m
  Transform1 : sm_lib/Frames and Transforms/Rigid Transform  RequirementInfo={} %GIDa_acd77a73_b388_4f92_9d7f_80455fcc6f03  RotationMethod=ArbitraryAxis  FollAlignAxisA=+X  BaseAlignAxisA=+Y  FollAlignAxisB=+Y  BaseAlignAxisB=+Z  RotationStandardAxis=+Z  RotationAngle=smiData.RigidTransform(179).angle  RotationAngleUnits=rad  RotationArbitraryAxis=smiData.RigidTransform(179).axis  RotationSequenceAxes=FollowerAxes  RotationSequence=XYX  RotationSequenceAngles=[0 0 0]  RotationSequenceAnglesUnits=deg  RotationMatrix=[1 0 0; 0 1 0; 0 0 1]  Quaternion=[1 0 0 0]  TranslationMethod=Cartesian  TranslationCartesianOffset=smiData.RigidTransform(179).translation  TranslationCartesianOffsetUnits=m  TranslationStandardAxis=+Z  TranslationStandardOffset=0  TranslationStandardOffsetUnits=m  TranslationROffset=0  TranslationROffsetUnits=m  TranslationThetaOffset=0  TranslationThetaOffsetUnits=deg  TranslationZOffset=0  TranslationZOffsetUnits=m
  G : PMIOPort  RequirementInfo={} %GIDa_0db8e743_6263_4cb7_8c42_12a083e85b55  Side=Left
  F : PMIOPort  RequirementInfo={} %GIDa_3ffddf9b_9544_486f_802d_b9754e064a1a  Port=2  Side=Right
  connections:
  Transform Manual4Vis/LConn1 -- ReferenceFrame/RConn1 -- Transform1/LConn1 -- Transform/RConn1
  Transform/LConn1 -- G/RConn1
  Transform1/RConn1 -- F/RConn1
  Transform Manual4Vis/RConn1 -- Solid/RConn1

== system sm_aileron_actuator_mech_01_ail/Aileron_Att_1/MountR_Att_1/Bracket L/Bolt LBrk ==
  Hex_Bolt_M10_1_RIGID : Subsystem  RequirementInfo={} %GIDa_29ce5607_ae7f_4d35_a262_73aea78fda16
  Washer_1_RIGID : Subsystem  RequirementInfo={} %GIDa_b3b32eee_c1ba_412b_bf70_78abf0e817cc
  B : PMIOPort  RequirementInfo={} %GIDa_f435952b_11a3_47b8_ac58_d7cc3fca700e  Side=Left
  connections:
  B/RConn1 -- Washer_1_RIGID/LConn1 -- Hex_Bolt_M10_1_RIGID/LConn1

== system sm_aileron_actuator_mech_01_ail/Aileron_Att_1/MountR_Att_1/Bracket L/Screws LBrk ==
  Oval_Head_M4_10_RIGID : Subsystem  RequirementInfo={} %GIDa_56cd4de4_e4e5_4d43_8df4_f7f74507892c
  Oval_Head_M4_11_RIGID : Subsystem  RequirementInfo={} %GIDa_0403a841_ef61_495b_a36f_e3ed77709937
  Oval_Head_M4_12_RIGID : Subsystem  RequirementInfo={} %GIDa_5643ca42_002d_4317_9aeb_99c0a0783509
  Oval_Head_M4_5_RIGID : Subsystem  RequirementInfo={} %GIDa_895f0917_b9ae_4ddf_a951_1e74619e936f
  Oval_Head_M4_6_RIGID : Subsystem  RequirementInfo={} %GIDa_b99e630b_7594_4d45_a314_f91642b8a534
  Oval_Head_M4_8_RIGID : Subsystem  RequirementInfo={} %GIDa_1d312c3b_549a_4985_865e_33cc40417e93
  B : PMIOPort  RequirementInfo={} %GIDa_45242911_4ba9_4372_aad2_d305e8b74db8  Side=Left
  connections:
  Oval_Head_M4_10_RIGID/LConn1 -- Oval_Head_M4_12_RIGID/LConn1 -- Oval_Head_M4_11_RIGID/LConn1 -- Oval_Head_M4_5_RIGID/LConn1 -- Oval_Head_M4_6_RIGID/LConn1 -- Oval_Head_M4_8_RIGID/LConn1 -- B/RConn1

== system sm_aileron_actuator_mech_01_ail/Aileron_Att_1/MountR_Att_1/Bracket R/AilBrk_R_1_RIGID ==
  ReferenceFrame : sm_lib/Frames and Transforms/Reference Frame  RequirementInfo={} %GIDa_13420bda_01d8_4041_867c_ad741a43369c
  Solid : sm_lib/Body Elements/File Solid  RequirementInfo={} %GIDa_2f5223d6_d3b6_400e_b97e_8e8cd782c40a  ExtGeomFileName=AilBrk_R.step  UnitType=FromFile  ExtGeomFileUnits=m  StepReaderType=HEX  ExportConvexHullGeometry=off  InertiaType=Custom  BasedOnType=Density  Density=1000  DensityUnits=kg/m^3  Mass=smiData.Solid(16).mass  MassUnits=kg  CenterOfMass=smiData.Solid(16).CoM  CenterOfMassUnits=m  MomentsOfInertia=smiData.Solid(16).MoI  MomentsOfInertiaUnits=kg*m^2  ProductsOfInertia=smiData.Solid(16).PoI  ProductsOfInertiaUnits=kg*m^2  GraphicType=FromGeometry  MarkerShape=Sphere  MarkerSize=10  GraphicVisPropType=SimpleVisualProperties  GraphicDiffuseColor=smiData.Solid(16).color  GraphicOpacity=smiData.Solid(16).opacity  GraphicSpecularColor=[0.5 0.5 0.5 1.0]  GraphicAmbientColor=[0.15 0.15 0.15 1.0]  GraphicEmissiveColor=[0.0 0.0 0.0 1.0]  GraphicShininess=75  DoExposeReferenceFrame=on  SerializedFrames=<Frames/>
  Transform : sm_lib/Frames and Transforms/Rigid Transform  RequirementInfo={} %GIDa_969d3219_0b38_469b_a17c_297ac23138c6  RotationMethod=ArbitraryAxis  FollAlignAxisA=+X  BaseAlignAxisA=+Y  FollAlignAxisB=+Y  BaseAlignAxisB=+Z  RotationStandardAxis=+Z  RotationAngle=smiData.RigidTransform(120).angle  RotationAngleUnits=rad  RotationArbitraryAxis=smiData.RigidTransform(120).axis  RotationSequenceAxes=FollowerAxes  RotationSequence=XYX  RotationSequenceAngles=[0 0 0]  RotationSequenceAnglesUnits=deg  RotationMatrix=[1 0 0; 0 1 0; 0 0 1]  Quaternion=[1 0 0 0]  TranslationMethod=Cartesian  TranslationCartesianOffset=smiData.RigidTransform(120).translation  TranslationCartesianOffsetUnits=m  TranslationStandardAxis=+Z  TranslationStandardOffset=0  TranslationStandardOffsetUnits=m  TranslationROffset=0  TranslationROffsetUnits=m  TranslationThetaOffset=0  TranslationThetaOffsetUnits=deg  TranslationZOffset=0  TranslationZOffsetUnits=m
  Transform Manual4Vis : sm_lib/Frames and Transforms/Rigid Transform  RequirementInfo={} %GIDa_ded112bd_2a9d_46a2_83bc_15371b6ba78a  RotationMethod=None  FollAlignAxisA=+X  BaseAlignAxisA=+Y  FollAlignAxisB=+Y  BaseAlignAxisB=+Z  RotationStandardAxis=+Z  RotationAngle=0.0  RotationAngleUnits=deg  RotationArbitraryAxis=[0 0 1]  RotationSequenceAxes=FollowerAxes  RotationSequence=XYX  RotationSequenceAngles=[0 0 0]  RotationSequenceAnglesUnits=deg  RotationMatrix=[1 0 0; 0 1 0; 0 0 1]  Quaternion=[1 0 0 0]  TranslationMethod=StandardAxis  TranslationCartesianOffset=[0 0 0]  TranslationCartesianOffsetUnits=m  TranslationStandardAxis=-Y  TranslationStandardOffset=AAC_Param.AilBrk.LRManual4Vis  TranslationStandardOffsetUnits=m  TranslationROffset=0  TranslationROffsetUnits=m  TranslationThetaOffset=0  TranslationThetaOffsetUnits=deg  TranslationZOffset=0  TranslationZOffsetUnits=m
  Transform1 : sm_lib/Frames and Transforms/Rigid Transform  RequirementInfo={} %GIDa_5e0bb33a_0a02_492c_ae3b_9e0557c90836  RotationMethod=ArbitraryAxis  FollAlignAxisA=+X  BaseAlignAxisA=+Y  FollAlignAxisB=+Y  BaseAlignAxisB=+Z  RotationStandardAxis=+Z  RotationAngle=smiData.RigidTransform(178).angle  RotationAngleUnits=rad  RotationArbitraryAxis=smiData.RigidTransform(178).axis  RotationSequenceAxes=FollowerAxes  RotationSequence=XYX  RotationSequenceAngles=[0 0 0]  RotationSequenceAnglesUnits=deg  RotationMatrix=[1 0 0; 0 1 0; 0 0 1]  Quaternion=[1 0 0 0]  TranslationMethod=Cartesian  TranslationCartesianOffset=smiData.RigidTransform(178).translation  TranslationCartesianOffsetUnits=m  TranslationStandardAxis=+Z  TranslationStandardOffset=0  TranslationStandardOffsetUnits=m  TranslationROffset=0  TranslationROffsetUnits=m  TranslationThetaOffset=0  TranslationThetaOffsetUnits=deg  TranslationZOffset=0  TranslationZOffsetUnits=m
  G : PMIOPort  RequirementInfo={} %GIDa_76d414ba_354f_48d4_bb23_42fb8a2de713  Side=Left
  F : PMIOPort  RequirementInfo={} %GIDa_efe6b5c1_1cc2_4f60_a1d4_87f961d79a39  Port=2  Side=Right
  connections:
  Transform Manual4Vis/RConn1 -- Solid/RConn1
  Transform/LConn1 -- G/RConn1
  Transform1/RConn1 -- F/RConn1
  Transform Manual4Vis/LConn1 -- ReferenceFrame/RConn1 -- Transform1/LConn1 -- Transform/RConn1

== system sm_aileron_actuator_mech_01_ail/Aileron_Att_1/MountR_Att_1/Bracket R/Bolt RBrk ==
  Hex_Bolt_M10_2_RIGID : Subsystem  RequirementInfo={} %GIDa_cea0b079_1283_435b_ba4b_b94c055c2fa6
  Washer_3_RIGID : Subsystem  RequirementInfo={} %GIDa_4934e7ef_fd32_4bf4_a86a_b22c4db0ce81
  G : PMIOPort  RequirementInfo={} %GIDa_4ed82da9_28b5_4e47_a202_c9623457144c  Side=Left
  connections:
  G/RConn1 -- Washer_3_RIGID/LConn1 -- Hex_Bolt_M10_2_RIGID/LConn1

== system sm_aileron_actuator_mech_01_ail/Aileron_Att_1/MountR_Att_1/Bracket R/Screws RBrk ==
  Oval_Head_M4_1_RIGID : Subsystem  RequirementInfo={} %GIDa_916efa0e_f664_47c7_a700_42bda76f365b
  Oval_Head_M4_2_RIGID : Subsystem  RequirementInfo={} %GIDa_741fce72_4701_4080_a51f_c1b555829d44
  Oval_Head_M4_3_RIGID : Subsystem  RequirementInfo={} %GIDa_bf9f5c4d_00f0_4bc2_978c_a8fe882b30c8
  Oval_Head_M4_4_RIGID : Subsystem  RequirementInfo={} %GIDa_a2b815ab_cf9b_4f5b_8c6d_5c986c22d0a1
  Oval_Head_M4_7_RIGID : Subsystem  RequirementInfo={} %GIDa_df0ed7d3_b75f_419f_abee_0f439acd86d0
  Oval_Head_M4_9_RIGID : Subsystem  RequirementInfo={} %GIDa_29ed9d3a_baf9_4abc_bfde_168044d1c30f
  G : PMIOPort  RequirementInfo={} %GIDa_6da213b4_8c72_4685_9e6e_780093ee071e  Side=Left
  connections:
  Oval_Head_M4_1_RIGID/LConn1 -- Oval_Head_M4_3_RIGID/LConn1 -- Oval_Head_M4_2_RIGID/LConn1 -- G/RConn1 -- Oval_Head_M4_9_RIGID/LConn1 -- Oval_Head_M4_7_RIGID/LConn1 -- Oval_Head_M4_4_RIGID/LConn1

== system sm_aileron_actuator_mech_01_ail/Aileron_Att_1/MountC_Att_1/Bracket C/Bolt CBrk/Hex_Flange_Screw_M6_1_RIGID ==
  ReferenceFrame : sm_lib/Frames and Transforms/Reference Frame  RequirementInfo={} %GIDa_7dffdcd6_527e_4a51_bdb5_504d4f12043e
  Solid : sm_lib/Body Elements/File Solid  RequirementInfo={} %GIDa_b2a4ab35_f782_4a84_888e_afabf2fff811  ExtGeomFileName=Hex_Flange_Screw_M6.step  UnitType=FromFile  ExtGeomFileUnits=m  StepReaderType=HEX  ExportConvexHullGeometry=off  InertiaType=Custom  BasedOnType=Density  Density=1000  DensityUnits=kg/m^3  Mass=smiData.Solid(11).mass  MassUnits=kg  CenterOfMass=smiData.Solid(11).CoM  CenterOfMassUnits=m  MomentsOfInertia=smiData.Solid(11).MoI  MomentsOfInertiaUnits=kg*m^2  ProductsOfInertia=smiData.Solid(11).PoI  ProductsOfInertiaUnits=kg*m^2  GraphicType=FromGeometry  MarkerShape=Sphere  MarkerSize=10  GraphicVisPropType=SimpleVisualProperties  GraphicDiffuseColor=smiData.Solid(11).color  GraphicOpacity=smiData.Solid(11).opacity  GraphicSpecularColor=[0.5 0.5 0.5 1.0]  GraphicAmbientColor=[0.15 0.15 0.15 1.0]  GraphicEmissiveColor=[0.0 0.0 0.0 1.0]  GraphicShininess=75  DoExposeReferenceFrame=on  SerializedFrames=<Frames/>
  Transform : sm_lib/Frames and Transforms/Rigid Transform  RequirementInfo={} %GIDa_e2edc983_9d0a_4de2_87f0_6c5bd699c093  RotationMethod=ArbitraryAxis  FollAlignAxisA=+X  BaseAlignAxisA=+Y  FollAlignAxisB=+Y  BaseAlignAxisB=+Z  RotationStandardAxis=+Z  RotationAngle=smiData.RigidTransform(99).angle  RotationAngleUnits=rad  RotationArbitraryAxis=smiData.RigidTransform(99).axis  RotationSequenceAxes=FollowerAxes  RotationSequence=XYX  RotationSequenceAngles=[0 0 0]  RotationSequenceAnglesUnits=deg  RotationMatrix=[1 0 0; 0 1 0; 0 0 1]  Quaternion=[1 0 0 0]  TranslationMethod=Cartesian  TranslationCartesianOffset=smiData.RigidTransform(99).translation  TranslationCartesianOffsetUnits=m  TranslationStandardAxis=+Z  TranslationStandardOffset=0  TranslationStandardOffsetUnits=m  TranslationROffset=0  TranslationROffsetUnits=m  TranslationThetaOffset=0  TranslationThetaOffsetUnits=deg  TranslationZOffset=0  TranslationZOffsetUnits=m
  G : PMIOPort  RequirementInfo={} %GIDa_1de79099_ab7d_4bd7_83f6_e841196a3c9c  Side=Left
  connections:
  Solid/RConn1 -- ReferenceFrame/RConn1 -- Transform/RConn1
  Transform/LConn1 -- G/RConn1

== system sm_aileron_actuator_mech_01_ail/Aileron_Att_1/MountC_Att_1/Bracket C/Bolt CBrk/Hex_Flange_Screw_M6_2_RIGID ==
  ReferenceFrame : sm_lib/Frames and Transforms/Reference Frame  RequirementInfo={} %GIDa_beb33409_0f04_431b_ae0d_3b2c6af2db1a
  Solid : sm_lib/Body Elements/File Solid  RequirementInfo={} %GIDa_5bd7eed4_b28c_464a_870d_253d835463e7  ExtGeomFileName=Hex_Flange_Screw_M6.step  UnitType=FromFile  ExtGeomFileUnits=m  StepReaderType=HEX  ExportConvexHullGeometry=off  InertiaType=Custom  BasedOnType=Density  Density=1000  DensityUnits=kg/m^3  Mass=smiData.Solid(11).mass  MassUnits=kg  CenterOfMass=smiData.Solid(11).CoM  CenterOfMassUnits=m  MomentsOfInertia=smiData.Solid(11).MoI  MomentsOfInertiaUnits=kg*m^2  ProductsOfInertia=smiData.Solid(11).PoI  ProductsOfInertiaUnits=kg*m^2  GraphicType=FromGeometry  MarkerShape=Sphere  MarkerSize=10  GraphicVisPropType=SimpleVisualProperties  GraphicDiffuseColor=smiData.Solid(11).color  GraphicOpacity=smiData.Solid(11).opacity  GraphicSpecularColor=[0.5 0.5 0.5 1.0]  GraphicAmbientColor=[0.15 0.15 0.15 1.0]  GraphicEmissiveColor=[0.0 0.0 0.0 1.0]  GraphicShininess=75  DoExposeReferenceFrame=on  SerializedFrames=<Frames/>
  Transform : sm_lib/Frames and Transforms/Rigid Transform  RequirementInfo={} %GIDa_31d27c49_f783_40c6_bbb2_be6b3a59b4f6  RotationMethod=ArbitraryAxis  FollAlignAxisA=+X  BaseAlignAxisA=+Y  FollAlignAxisB=+Y  BaseAlignAxisB=+Z  RotationStandardAxis=+Z  RotationAngle=smiData.RigidTransform(96).angle  RotationAngleUnits=rad  RotationArbitraryAxis=smiData.RigidTransform(96).axis  RotationSequenceAxes=FollowerAxes  RotationSequence=XYX  RotationSequenceAngles=[0 0 0]  RotationSequenceAnglesUnits=deg  RotationMatrix=[1 0 0; 0 1 0; 0 0 1]  Quaternion=[1 0 0 0]  TranslationMethod=Cartesian  TranslationCartesianOffset=smiData.RigidTransform(96).translation  TranslationCartesianOffsetUnits=m  TranslationStandardAxis=+Z  TranslationStandardOffset=0  TranslationStandardOffsetUnits=m  TranslationROffset=0  TranslationROffsetUnits=m  TranslationThetaOffset=0  TranslationThetaOffsetUnits=deg  TranslationZOffset=0  TranslationZOffsetUnits=m
  G : PMIOPort  RequirementInfo={} %GIDa_34617b27_cd3a_4875_a076_4d5f53fc3ee6  Side=Left
  connections:
  Solid/RConn1 -- ReferenceFrame/RConn1 -- Transform/RConn1
  Transform/LConn1 -- G/RConn1
